simulink library "lib_hysteresis_debounce"  (R2023a)
settings: Solver=VariableStepAuto  StartTime=0.0  StopTime=10.0  RelTol=1e-3
settings Model: Creator=YXQ1WX  LastModifiedBy=xiaoqiang.yuan
settings OptimizationCC: ReuseModelBlockBuffer=off

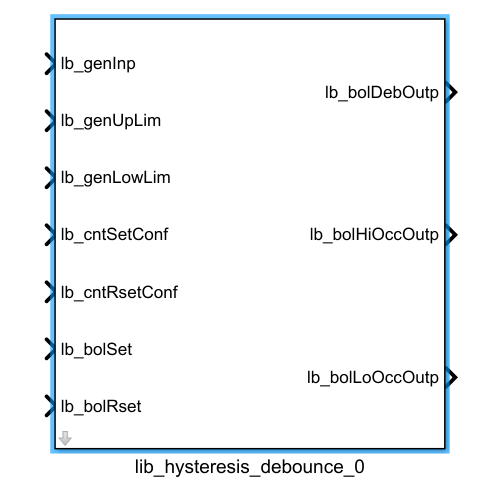
[thumbnail: Simulink's stored preview of the top-level diagram]
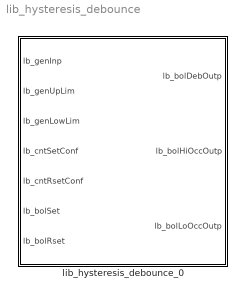
== system lib_hysteresis_debounce ==
  lib_hysteresis_debounce_0 : Subsystem  RTWFcnName=HysteresisDebounce  RTWFileName=VHIT_control_library  mask(Hysteresis){lb_parInitOutp=0}
      mask prompts: lb_parInitOutp "Initialization value:"
      mask help:
      | 1. x(k) < xLo:           y(k) = yLo;
      | 2. xLo ≤ x(k) ≤ xHi:   y(k) = y(k-1);
      | 3. x(k) > xHi:           y(k) = yHi.
      settings: RTWFcnNameOpts=User specified
      mask DialogControl DescGroupVar Prompt: VHIT control library
      mask DialogControl DescTextVar Prompt: For Hysteresis and Debounce

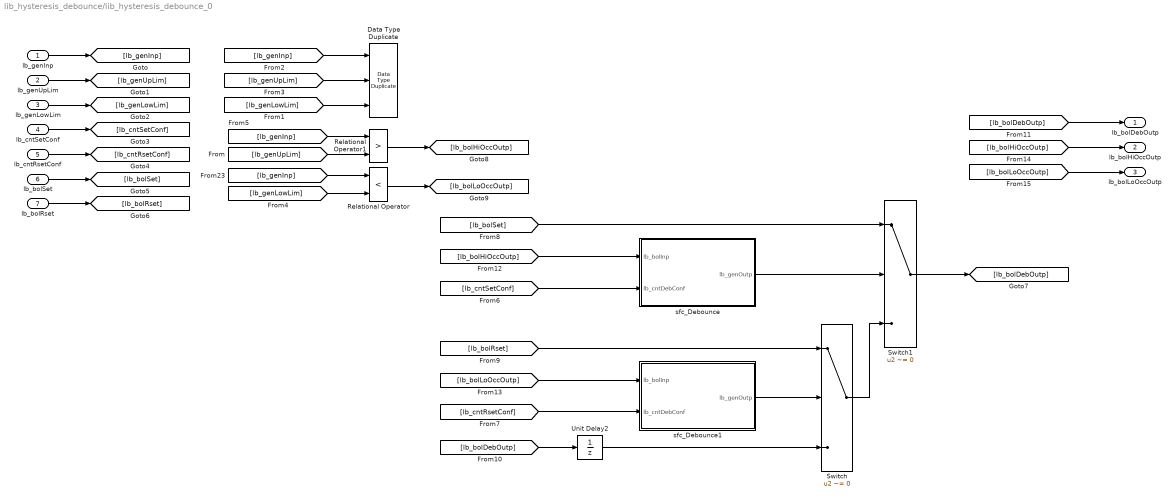
== system lib_hysteresis_debounce/lib_hysteresis_debounce_0 ==
  lb_genInp : Inport
  lb_genUpLim : Inport  Port=2
  lb_genLowLim : Inport  Port=3
  lb_cntSetConf : Inport  Port=4
  lb_cntRsetConf : Inport  Port=5
  lb_bolSet : Inport  Port=6
  lb_bolRset : Inport  Port=7
  Data Type Duplicate : DataTypeDuplicate  NumInputPorts=3
  Relational Operator : RelationalOperator  Operator=<  OutDataTypeStr=boolean  InputSameDT=off
  Relational Operator1 : RelationalOperator  Operator=>  OutDataTypeStr=boolean  InputSameDT=off
  Switch : Switch  Criteria=u2 ~= 0  SaturateOnIntegerOverflow=off  InputSameDT=off  OutDataTypeStr=Inherit: Same as first input
  Switch1 : Switch  Criteria=u2 ~= 0  SaturateOnIntegerOverflow=off  InputSameDT=off  OutDataTypeStr=Inherit: Same as first input
  Unit Delay2 : UnitDelay  InitialCondition=lb_parInitOutp  SampleTime=-1  HasFrameUpgradeWarning=on
      settings: AttributesFormatString=iy = %<X0>
  sfc_Debounce : Stateflow chart  TreatAsAtomicUnit=on
      settings: RTWSystemCode=Inline
  sfc_Debounce1 : Stateflow chart  TreatAsAtomicUnit=on
      settings: RTWSystemCode=Inline
  lb_bolDebOutp : Outport
  lb_bolHiOccOutp : Outport  Port=2
  lb_bolLoOccOutp : Outport  Port=3
  wires:
  [lb_genLowLim] -> Relational Operator/2
  [lb_genInp] -> Relational Operator/1
  Switch1/1 -> [lb_bolDebOutp]
  [lb_genUpLim] -> Relational Operator1/2
  [lb_cntSetConf] -> sfc_Debounce/2(lb_cntDebConf)
  lb_genInp/1 -> [lb_genInp]
  lb_genUpLim/1 -> [lb_genUpLim]
  lb_genLowLim/1 -> [lb_genLowLim]
  [lb_genInp] -> Data Type Duplicate/1
  [lb_genUpLim] -> Data Type Duplicate/2
  [lb_genLowLim] -> Data Type Duplicate/3
  [lb_genInp] -> Relational Operator1/1
  lb_cntSetConf/1 -> [lb_cntSetConf]
  lb_cntRsetConf/1 -> [lb_cntRsetConf]
  lb_bolSet/1 -> [lb_bolSet]
  sfc_Debounce/1(lb_genOutp) -> Switch1/2
  lb_bolRset/1 -> [lb_bolRset]
  Unit Delay2/1 -> Switch/3
  [lb_bolDebOutp] -> Unit Delay2/1
  sfc_Debounce1/1(lb_genOutp) -> Switch/2
  Switch/1 -> Switch1/3
  [lb_cntRsetConf] -> sfc_Debounce1/2(lb_cntDebConf)
  [lb_bolRset] -> Switch/1
  [lb_bolSet] -> Switch1/1
  [lb_bolDebOutp] -> lb_bolDebOutp/1
  Relational Operator1/1 -> [lb_bolHiOccOutp]
  Relational Operator/1 -> [lb_bolLoOccOutp]
  [lb_bolHiOccOutp] -> sfc_Debounce/1(lb_bolInp)
  [lb_bolLoOccOutp] -> sfc_Debounce1/1(lb_bolInp)
  [lb_bolHiOccOutp] -> lb_bolHiOccOutp/1
  [lb_bolLoOccOutp] -> lb_bolLoOccOutp/1

== stateflow chart lib_hysteresis_debounce/lib_hysteresis_debounce_0/sfc_Debounce1 ==
  state Wait
    en:  lb_cntDebCond = uint16(0);
    lb_genOutp = false;
  state Confirming
    /*Set Bit0*/
    en:lb_cntDebCond++;lb_genOutp = false;
    du:lb_cntDebCond++;
  state Confirm
    /*Set Bit0 Bit1*/
    en: lb_cntDebCond = uint16(0);lb_genOutp = true;
  (default) -> (junction 179)
  (junction 179) -> (junction 181) [order 1] : /*There is Fault*/
      | [lb_bolInp]
  (junction 181) -> (junction 184) [order 1] : /*Direct Confirm*/
      | [lb_cntDebConf == uint16(0)]
  (junction 179) -> Wait [order 2]
  (junction 181) -> Confirming [order 2]
  (junction 184) -> Confirm
  Confirming -> Wait [order 1] : /*There is no Fault*/
      | [!lb_bolInp]
  (junction 212) -> Confirming [order 2] : /*Need Debounce*/
  Wait -> (junction 212) : /*There is Fault*/
      | [lb_bolInp]
  (junction 212) -> Confirm [order 1] : /*Direct Confirm*/
      | [lb_cntDebConf == uint16(0)]
  Confirm -> Wait : /*There is no Fault*/
      | [!lb_bolInp]
  Confirming -> Confirm [order 2] : /*Fault Is Confirmed*/
      | [lb_cntDebCond >= lb_cntDebConf]
  data: lb_bolInp input boolean; lb_cntDebConf input uint16; lb_genOutp output boolean; lb_cntDebCond local uint16
  data lb_bolInp settings: description=$TL$ inheritscaling=1; $TL$
  data lb_cntDebConf settings: description=$TL$ inheritscaling=1; $TL$
  data lb_genOutp settings: description=$TL$ type=UInt8; $TL$
  data lb_cntDebCond settings: description=$TL$ type=UInt16; $TL$

== stateflow chart lib_hysteresis_debounce/lib_hysteresis_debounce_0/sfc_Debounce ==
  state Wait
    en:  lb_cntDebCond = uint16(0);
    lb_genOutp = false;
  state Confirming
    /*Set Bit0*/
    en:lb_cntDebCond++;lb_genOutp = false;
    du:lb_cntDebCond++;
  state Confirm
    /*Set Bit0 Bit1*/
    en: lb_cntDebCond = uint16(0);lb_genOutp = true;
  (default) -> (junction 179)
  (junction 179) -> (junction 181) [order 1] : /*There is Fault*/
      | [lb_bolInp]
  (junction 181) -> (junction 184) [order 1] : /*Direct Confirm*/
      | [lb_cntDebConf == uint16(0)]
  (junction 179) -> Wait [order 2]
  (junction 181) -> Confirming [order 2]
  (junction 184) -> Confirm
  Confirming -> Wait [order 1] : /*There is no Fault*/
      | [!lb_bolInp]
  (junction 212) -> Confirming [order 2] : /*Need Debounce*/
  Wait -> (junction 212) : /*There is Fault*/
      | [lb_bolInp]
  (junction 212) -> Confirm [order 1] : /*Direct Confirm*/
      | [lb_cntDebConf == uint16(0)]
  Confirm -> Wait : /*There is no Fault*/
      | [!lb_bolInp]
  Confirming -> Confirm [order 2] : /*Fault Is Confirmed*/
      | [lb_cntDebCond >= lb_cntDebConf]
  data: lb_bolInp input boolean; lb_cntDebConf input uint16; lb_genOutp output boolean; lb_cntDebCond local uint16
  data lb_bolInp settings: description=$TL$ inheritscaling=1; $TL$
  data lb_cntDebConf settings: description=$TL$ inheritscaling=1; $TL$
  data lb_genOutp settings: description=$TL$ type=UInt8; $TL$
  data lb_cntDebCond settings: description=$TL$ type=UInt16; $TL$
